simulink model "CA - Linear - Simulink"  (R2022b)
settings: Solver=VariableStepAuto  StartTime=0.0  StopTime=500  RelTol=1e-3
libraries: simulink x2
settings Model: Creator=SHAHAB  LastModifiedBy=SHAHAB

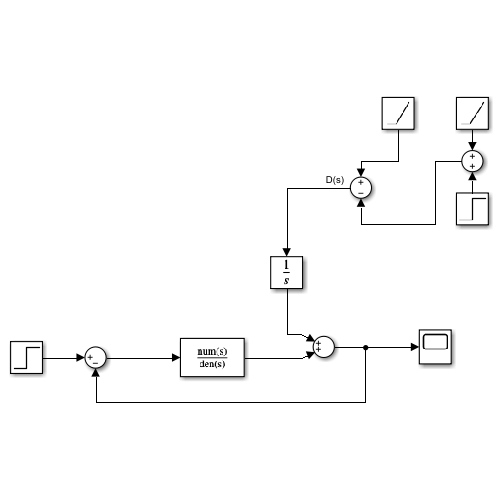
[thumbnail: Simulink's stored preview of the top-level diagram]
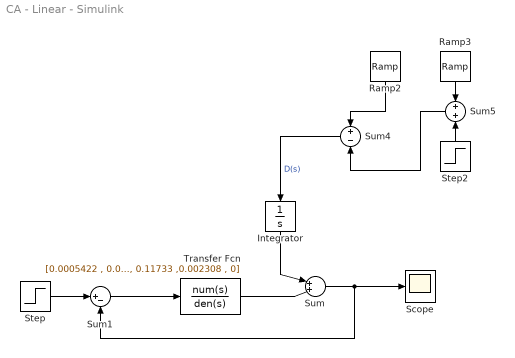
== system CA - Linear - Simulink ==
  Integrator : Integrator
  Ramp2 : simulink/Sources/Ramp  slope=0.5  start=0  InitialOutput=0
  Ramp3 : simulink/Sources/Ramp  slope=0.5  start=1  InitialOutput=0
  Scope : Scope
  Step : Step  Time=0  SampleTime=500
  Step2 : Step  After=0.5  SampleTime=1
  Sum : Sum  Inputs=|++|
  Sum1 : Sum  Inputs=|+-
  Sum4 : Sum  Inputs=+-
  Sum5 : Sum
  Transfer Fcn : TransferFcn  Numerator=[0.0005422 , 0.00003116]  Denominator=[1 , 0.11733 ,0.002308 , 0]
  wires:
  Step2/1 -> Sum5/2
  Ramp3/1 -> Sum5/1
  Ramp2/1 -> Sum4/1
  Sum5/1 -> Sum4/2
  Step/1 -> Sum1/1
  Sum1/1 -> Transfer Fcn/1
  Transfer Fcn/1 -> Sum/2
  Sum/1 -> Sum1/2, Scope/1
  Sum4/1 -> Integrator/1  "D(s)"
  Integrator/1 -> Sum/1
